simulink model "CCO_DSM_RDAC_02"  (R2021a)
settings: Solver=VariableStepAuto  StartTime=0.0  StopTime=6000*clk_p  RelTol=1e-3
values from neighbouring files (symbols this model uses):
  clk_p = 1/clk    (= 5e-09)    [parallel_simulink_test8.m]
  finw = 2*pi*M/(N_in*clk_p)    (= 3374757.73335)    [parallel_simulink_test8.m]
  N = 31    [GradientD_v6.m]    (also in N_selection.m = ceil(N); front_end_syn.m = input('How many stages of quantizer (enter num)? '); parallel_simulink_test8.m = 27; power_esti_v1.m)
  N_stage = N    (= 27)    [parallel_simulink_test8.m]
  Ph2 = circshift(Ph, (N_stage+1)/2)    [parallel_simulink_test8.m]
  Ru = VDD/(kdac*1e-6) - (Rcco*VDD*N)/(2*Amp) - N*Rcco    [solve_param_2nd.m]    (also in solve_param_2nd_1st.m; solve_param_RDAC_N_v5.m; solve_param_RDAC_N_v6.m; solve_param_comb_v1.m)
  S = 5    [GradientD_v6.m]    (also in parallel_simulink_test8.m; power_esti_v1.m; solve_param_2nd.m; solve_param_2nd_1st.m = 1)
  VDD = 1.2    [power_esti_v1.m]    (also in solve_param_2nd.m; solve_param_2nd_1st.m; solve_param_RDAC_N_v5.m; solve_param_RDAC_N_v6.m)
undefined symbols (not defined in the file or in its folder): Amp_in, Bias, Compen, fix_valid, gain_DAC, kcco_gain, Ph, Res, Res_CCO_fix
libraries: commblksprivate x4, simulink_extras x3, dspsigattribs x2, commsynccomp2 x2, simulink x1
settings Model: SimulationMode=accelerator  OrderedModelArguments=off  Creator=97826  LastModifiedBy=kli416
settings SolverCC: AlgebraicLoopSolver=LineSearch
settings DebuggingCC: SFMachineParentedDataDiag=warning
settings SFSimCC: CustomCodeUndefinedFunction=UseInterfaceOnly

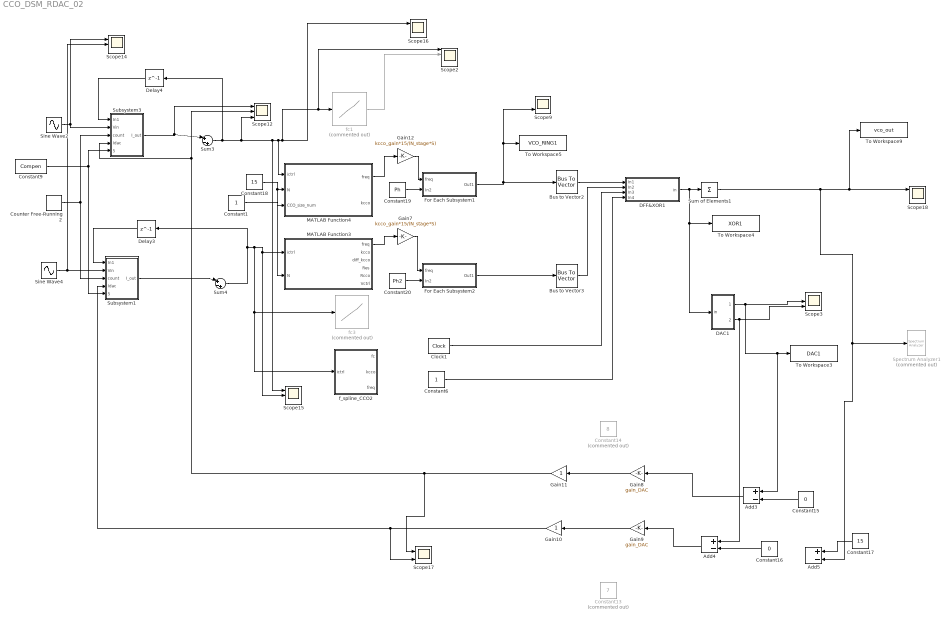
== system CCO_DSM_RDAC_02 ==
  Add3 : Sum  Inputs=+-
  Add4 : Sum  Inputs=+-
  Add5 : Sum  Inputs=+-
  Bus to Vector2 : BusToVector
  Bus to Vector3 : BusToVector
  Clock1 : simulink_extras/Flip Flops/Clock  period=clk_p
  Constant1 : Constant  VectorParams1D=off
  Constant13 : Constant  Commented=on  Value=7
  Constant14 : Constant  Commented=on  Value=8
  Constant15 : Constant  Value=0
  Constant16 : Constant  Value=0
  Constant17 : Constant  Value=15
  Constant18 : Constant  Value=15  VectorParams1D=off
  Constant19 : Constant  Value=Ph  VectorParams1D=off
  Constant20 : Constant  Value=Ph2  VectorParams1D=off
  Constant6 : Constant
  Constant9 : Constant  Value=Compen
  Counter Free-Running2 : simulink/Sources/Counter Free-Running  NumBits=32  tsamp=clk_p
  DAC1 : Subsystem
  DFF&XOR1 : Subsystem  TreatAsAtomicUnit=on
  Delay3 : Delay  DelayLength=1  SampleTime=clk_p
  Delay4 : Delay  DelayLength=1  SampleTime=clk_p
  For Each Subsystem1 : Subsystem  TreatAsAtomicUnit=on
  For Each Subsystem2 : Subsystem  TreatAsAtomicUnit=on
  Gain10 : Gain
  Gain11 : Gain
  Gain12 : Gain  Gain=kcco_gain*15/(N_stage*S)
  Gain7 : Gain  Gain=kcco_gain*15/(N_stage*S)
  Gain8 : Gain  Gain=gain_DAC
  Gain9 : Gain  Gain=gain_DAC
  MATLAB Function3 : MATLAB Function  TreatAsAtomicUnit=on
  MATLAB Function4 : MATLAB Function  TreatAsAtomicUnit=on
  Scope{3,12,14..16,18} (6 alike) : Scope  NumInputPorts=3
  Scope17 : Scope  NumInputPorts=2
  Scope2 : Scope  NumInputPorts=4
  Scope9 : Scope  NumInputPorts=2
  Sine Wave2 : Sin  Amplitude=Amp_in  Bias=Bias  Frequency=finw  SampleTime=0
  Sine Wave4 : Sin  Amplitude=Amp_in  Bias=Bias  Frequency=finw  Phase=pi  SampleTime=0
  Spectrum Analyzer1 : SpectrumAnalyzer  Commented=on
  Subsystem1 : Subsystem
  Subsystem3 : Subsystem
  Sum of Elements1 : Sum  Inputs=+  CollapseMode=Specified dimension
  Sum3 : Sum  Inputs=|+-+
  Sum4 : Sum  Inputs=|+-+
  To Workspace3 : ToWorkspace  VariableName=DAC1  SampleTime=-1
  To Workspace4 : ToWorkspace  VariableName=XOR1  SampleTime=-1
  To Workspace5 : ToWorkspace  VariableName=VCO_RING1  SampleTime=-1
  To Workspace9 : ToWorkspace  VariableName=vco_out  SampleTime=-1
  f_spline_CCO2 : MATLAB Function  TreatAsAtomicUnit=on
  fc1 : Lookup_n-D  Commented=on  NumberOfTableDimensions=1  BreakpointsForDimension1="[0.2, 0.3, 0.4, 0.5, 0.6, 0.7, 0.8, 0.9, 1.0, 1.1, 1.2, 1.3, 1.4, 1.5, 1.6, 1.7, 1.8, 1.9, 2, 3, 4, 5, 6, 7, 8, 9, 10, 15, 20, 25, 30, 35, 40, 45, 50, 55,  60, 65,  70, 75, 80, 85, 90, 95,  100, 105, 110, 115, 120, 125,  130, 135, 140, 145, 150, 155, 160, 165, 170, 175, 180, 185, 190, 195, 200]"  Table=|  InternalRulePriority=Speed  RndMeth=Simplest  InputSameDT=on
      | [1.66447511e+06, 2.39120610e+06, 3.09209814e+06, 3.77442525e+06,...
      |        4.44233187e+06, 5.09847708e+06, 5.74468330e+06, 6.38231333e+06,...
      |        7.01222933e+06, 7.63545294e+06, 8.25259544e+06, 8.86438379e+06,...
      |        9.47104229e+06, 1.00727251e+07, 1.06702063e+07, 1.12634810e+07,...
      |        1.18529335e+07, 1.24387856e+07, 1.30211555e+07, 1.86896325e+07,...
      |        2.41398372e+07, 2.94282099e+07, 3.45871163e+07, 3.96389683e+07,...
      |        4.45976622e+07, 4.94748247e+07, 5.42802707e+07, 7.74257487e+07,...
      |        9.94391631e+07, 1.20601948e+08, 1.41072774e+08, 1.60965277e+08,...
      |        1.80356637e+08, 1.99308797e+08, 2.17870620e+08, 2.36073995e+08,...
      |        2.53954710e+08, 2.71542852e+08, 2.88847872e+08, 3.05898332e+08,...
      |        3.22708688e+08, 3.39290137e+08, 3.55660515e+08, 3.71827383e+08,...
      |        3.87804329e+08, 4.03598484e+08, 4.19215145e+08, 4.34671106e+08,...
      |        4.49972102e+08, 4.65109789e+08, 4.80106776e+08, 4.94966194e+08,...
      |        5.09681398e+08, 5.24271132e+08, 5.38732148e+08, 5.53069814e+08,...
      |        5.67288983e+08, 5.81395349e+08, 5.95390487e+08, 6.09269425e+08,...
      |        6.23056841e+08, 6.36731783e+08, 6.50300764e+08, 6.63790242e+08,...
      |        6.77167274e+08]
  fc3 : Lookup_n-D  Commented=on  NumberOfTableDimensions=1  BreakpointsForDimension1="[0.2, 0.3, 0.4, 0.5, 0.6, 0.7, 0.8, 0.9, 1.0, 1.1, 1.2, 1.3, 1.4, 1.5, 1.6, 1.7, 1.8, 1.9, 2, 3, 4, 5, 6, 7, 8, 9, 10, 15, 20, 25, 30, 35, 40, 45, 50, 55,  60, 65,  70, 75, 80, 85, 90, 95,  100, 105, 110, 115, 120, 125,  130, 135, 140, 145, 150, 155, 160, 165, 170, 175, 180, 185, 190, 195, 200]"  Table=|  InternalRulePriority=Speed  RndMeth=Simplest  InputSameDT=on
      | [1.66447511e+06, 2.39120610e+06, 3.09209814e+06, 3.77442525e+06,...
      |        4.44233187e+06, 5.09847708e+06, 5.74468330e+06, 6.38231333e+06,...
      |        7.01222933e+06, 7.63545294e+06, 8.25259544e+06, 8.86438379e+06,...
      |        9.47104229e+06, 1.00727251e+07, 1.06702063e+07, 1.12634810e+07,...
      |        1.18529335e+07, 1.24387856e+07, 1.30211555e+07, 1.86896325e+07,...
      |        2.41398372e+07, 2.94282099e+07, 3.45871163e+07, 3.96389683e+07,...
      |        4.45976622e+07, 4.94748247e+07, 5.42802707e+07, 7.74257487e+07,...
      |        9.94391631e+07, 1.20601948e+08, 1.41072774e+08, 1.60965277e+08,...
      |        1.80356637e+08, 1.99308797e+08, 2.17870620e+08, 2.36073995e+08,...
      |        2.53954710e+08, 2.71542852e+08, 2.88847872e+08, 3.05898332e+08,...
      |        3.22708688e+08, 3.39290137e+08, 3.55660515e+08, 3.71827383e+08,...
      |        3.87804329e+08, 4.03598484e+08, 4.19215145e+08, 4.34671106e+08,...
      |        4.49972102e+08, 4.65109789e+08, 4.80106776e+08, 4.94966194e+08,...
      |        5.09681398e+08, 5.24271132e+08, 5.38732148e+08, 5.53069814e+08,...
      |        5.67288983e+08, 5.81395349e+08, 5.95390487e+08, 6.09269425e+08,...
      |        6.23056841e+08, 6.36731783e+08, 6.50300764e+08, 6.63790242e+08,...
      |        6.77167274e+08]
  wires:
  Delay3/1 -> Subsystem1/1(In1)
  Sine Wave2/1 -> Subsystem3/2(Vin), Scope14/1
  Add4/1 -> Gain9/1
  Gain12/1 -> For Each Subsystem1/1(freq)
  Constant9/1 -> Subsystem1/5(compen), Subsystem3/5(compen)
  Sum4/1 -> Delay3/1, Scope15/2, MATLAB Function3/1(ictrl), f_spline_CCO2/1(ictrl), fc3/1
  Delay4/1 -> Subsystem3/1(In1)
  Sum of Elements1/1 -> Spectrum Analyzer1/1, Add5/2, Scope18/1, To Workspace9/1
  Sum3/1 -> Delay4/1, Scope12/3, Scope15/1, MATLAB Function4/1(ictrl), Scope2/1, fc1/1, Scope16/1
  Subsystem3/1(I_out) -> Scope12/1, Sum3/1
  Constant19/1 -> For Each Subsystem1/2(In2)
  Bus to Vector2/1 -> DFF&XOR1/1(In1)
  fc1/1 -> Scope2/2
  Counter Free-Running2/1 -> Subsystem1/3(count), Subsystem3/3(count)
  DAC1/2(out2) -> Add4/1, Scope3/3
  Constant16/1 -> Add4/2
  Constant6/1 -> DFF&XOR1/4(In4)
  Gain8/1 -> Gain11/1
  Gain10/1 -> Subsystem1/4(Idac), Scope17/2
  Constant18/1 -> MATLAB Function3/2(N), MATLAB Function4/2(N)
  Gain7/1 -> For Each Subsystem2/1(freq)
  Constant17/1 -> Add5/1
  Constant20/1 -> For Each Subsystem2/2(In2)
  DAC1/1(out1) -> Add3/1, To Workspace3/1, Scope3/2
  Gain9/1 -> Gain10/1
  Clock1/1 -> DFF&XOR1/3(In3)
  Constant15/1 -> Add3/2
  DFF&XOR1/1(in) -> To Workspace4/1, DAC1/1(in), Sum of Elements1/1
  Subsystem1/1(I_out) -> Sum4/1
  Bus to Vector3/1 -> DFF&XOR1/2(In2)
  For Each Subsystem2/1(Out1) -> Bus to Vector3/1
  Sine Wave4/1 -> Subsystem1/2(Vin), Scope14/2
  For Each Subsystem1/1(Out1) -> To Workspace5/1, Scope9/2, Bus to Vector2/1
  Add3/1 -> Gain8/1
  Gain11/1 -> Subsystem3/4(Idac), Scope12/2, Scope17/1
  MATLAB Function3/1(freq) -> Gain7/1
  MATLAB Function4/1(freq) -> Gain12/1
  Constant1/1 -> MATLAB Function4/3(CCO_size_num)

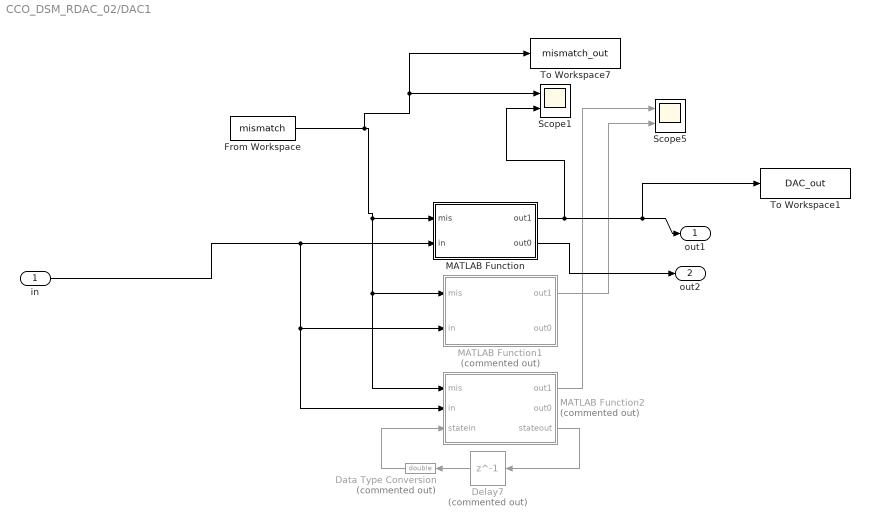
== system CCO_DSM_RDAC_02/DAC1 ==
  in : Inport
  Data Type Conversion : DataTypeConversion  Commented=on  OutDataTypeStr=double
  Delay7 : Delay  Commented=on  DelayLength=1  SampleTime=clk_p
  From Workspace : FromWorkspace  VariableName=mismatch
  MATLAB Function : MATLAB Function  TreatAsAtomicUnit=on
  MATLAB Function1 : MATLAB Function  Commented=on  TreatAsAtomicUnit=on
  MATLAB Function2 : MATLAB Function  Commented=on  TreatAsAtomicUnit=on
  Scope1 : Scope  NumInputPorts=2
  Scope5 : Scope  NumInputPorts=2
  To Workspace1 : ToWorkspace  VariableName=DAC_out  SampleTime=-1
  To Workspace7 : ToWorkspace  VariableName=mismatch_out  SampleTime=-1
  out1 : Outport
  out2 : Outport  Port=2
  wires:
  From Workspace/1 -> To Workspace7/1, Scope1/1, MATLAB Function2/1(mis), MATLAB Function1/1(mis), MATLAB Function/1(mis)
  MATLAB Function1/1(out1) -> Scope5/2
  MATLAB Function2/1(out1) -> Scope5/1
  MATLAB Function2/3(stateout) -> Delay7/1
  Delay7/1 -> Data Type Conversion/1
  Data Type Conversion/1 -> MATLAB Function2/3(statein)
  MATLAB Function/1(out1) -> Scope1/2, To Workspace1/1, out1/1
  MATLAB Function/2(out0) -> out2/1
  in/1 -> MATLAB Function2/2(in), MATLAB Function1/2(in), MATLAB Function/2(in)

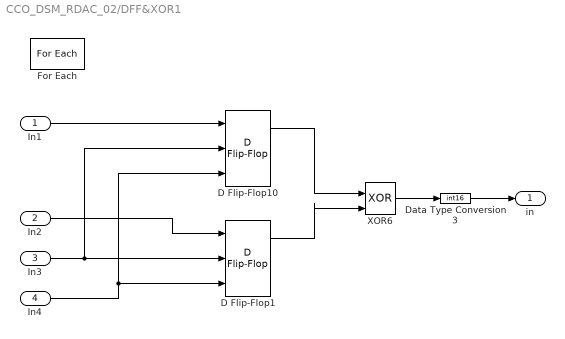
== system CCO_DSM_RDAC_02/DFF&XOR1 ==
  In1 : Inport  Partition=on  PartitionDimension=1  PartitionWidth=N_stage  PartitionOffset=0
  In2 : Inport  Port=2  Partition=on  PartitionDimension=1  PartitionWidth=N_stage  PartitionOffset=0
  In3 : Inport  Port=3
  In4 : Inport  Port=4
  D Flip-Flop1 : simulink_extras/Flip Flops/D Flip-Flop
  D Flip-Flop10 : simulink_extras/Flip Flops/D Flip-Flop
  Data Type Conversion3 : DataTypeConversion  OutDataTypeStr=int16
  For Each : ForEach  DisableCoverage=on
  XOR6 : Logic  Operator=XOR  IconShape=distinctive  AllPortsSameDT=off  OutDataTypeStr=boolean
  in : Outport  ConcatenationDimension=1
  wires:
  In1/1 -> D Flip-Flop10/1
  In3/1 -> D Flip-Flop1/2, D Flip-Flop10/2
  In4/1 -> D Flip-Flop1/3, D Flip-Flop10/3
  In2/1 -> D Flip-Flop1/1
  D Flip-Flop10/1 -> XOR6/1
  D Flip-Flop1/1 -> XOR6/2
  XOR6/1 -> Data Type Conversion3/1
  Data Type Conversion3/1 -> in/1

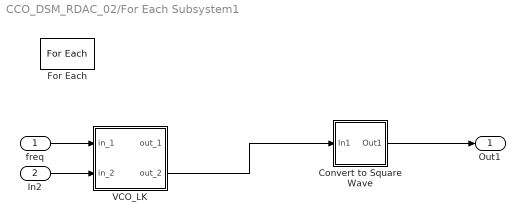
== system CCO_DSM_RDAC_02/For Each Subsystem1 ==
  freq : Inport
  In2 : Inport  Port=2  Partition=on  PartitionDimension=1  PartitionWidth=1  PartitionOffset=0
  Convert to Square Wave : Subsystem
  For Each : ForEach  DisableCoverage=on
  VCO_LK : Subsystem  mask{Ac=1, Fc=1, Kc=1, Ph=1}
  Out1 : Outport  ConcatenationDimension=1
  wires:
  freq/1 -> VCO_LK/1(in_1)
  Convert to Square Wave/1(Out1) -> Out1/1
  VCO_LK/2(out_2) -> Convert to Square Wave/1(In1)
  In2/1 -> VCO_LK/2(in_2)

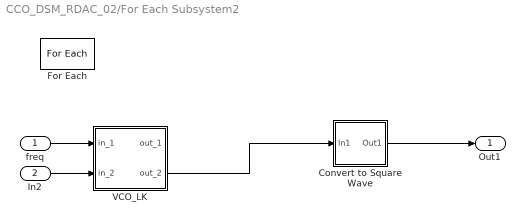
== system CCO_DSM_RDAC_02/For Each Subsystem2 ==
  freq : Inport
  In2 : Inport  Port=2  Partition=on  PartitionDimension=1  PartitionWidth=1  PartitionOffset=0
  Convert to Square Wave : Subsystem
  For Each : ForEach  DisableCoverage=on
  VCO_LK : Subsystem  mask{Ac=1, Fc=1, Kc=1, Ph=1}
  Out1 : Outport  ConcatenationDimension=1
  wires:
  freq/1 -> VCO_LK/1(in_1)
  Convert to Square Wave/1(Out1) -> Out1/1
  VCO_LK/2(out_2) -> Convert to Square Wave/1(In1)
  In2/1 -> VCO_LK/2(in_2)

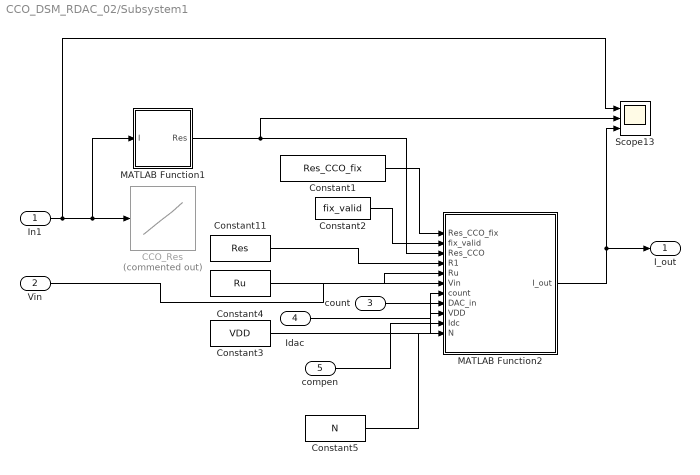
== system CCO_DSM_RDAC_02/Subsystem1 ==
  In1 : Inport
  Vin : Inport  Port=2
  count : Inport  Port=3
  Idac : Inport  Port=4
  compen : Inport  Port=5
  CCO_Res : Lookup_n-D  Commented=on  NumberOfTableDimensions=1  BreakpointsForDimension1="[0.2, 0.3, 0.4, 0.5, 0.6, 0.7, 0.8, 0.9, 1.0, 1.1, 1.2, 1.3, 1.4, 1.5, 1.6, 1.7, 1.8, 1.9, 2, 3, 4, 5, 6, 7, 8, 9, 10, 15, 20, 25, 30, 35, 40, 45, 50, 55,  60, 65,  70, 75, 80, 85, 90, 95,  100, 105, 110, 115, 120, 125,  130, 135, 140, 145, 150, 155, 160, 165, 170, 175, 180, 185, 190, 195, 200]"  Table=|  InternalRulePriority=Speed  RndMeth=Simplest  InputSameDT=on
      | [1537660.  , 1077280.  ,  842821.  ,  698885.  ,  591175.  ,...
      |         514638.  ,  459534.  ,  412343.  ,  375823.  ,  346689.  ,...
      |         319079.  ,  297528.  ,  279608.  ,  262772.  ,  247488.  ,...
      |         234050.  ,  222561.  ,  212364.  ,  203057.  ,  141281.  ,...
      |         109313.  ,   89599.1 ,   76189.9 ,   66472.9 ,   58960.7 ,...
      |          53105.2 ,   48293.7 ,   33792.1 ,   26194.2 ,   21517.8 ,...
      |          18368.6 ,   16013.  ,   14184.9 ,   12812.5 ,   11686.2 ,...
      |          10767.2 ,    9950.94,    9274.88,    8702.95,    8196.31,...
      |           7752.34,    7370.14,    7028.82,    6691.36,    6410.4 ,...
      |           6146.98,    5908.61,    5682.79,    5493.1 ,    5296.82,...
      |           5117.51,    4962.31,    4815.99,    4677.93,    4545.02,...
      |           4420.64,    4304.52,    4195.05,    4089.12,    3988.32,...
      |           3892.26,    3805.99,    3726.36,    3645.09,    3564.56]
  Constant1 : Constant  Value=Res_CCO_fix
  Constant11 : Constant  Value=Res
  Constant2 : Constant  Value=fix_valid
  Constant3 : Constant  Value=VDD
  Constant4 : Constant  Value=Ru
  Constant5 : Constant  Value=N
  MATLAB Function1 : MATLAB Function  TreatAsAtomicUnit=on
  MATLAB Function2 : MATLAB Function  TreatAsAtomicUnit=on
  Scope13 : Scope  NumInputPorts=3
  I_out : Outport
  wires:
  Constant11/1 -> MATLAB Function2/4(R1)
  Vin/1 -> MATLAB Function2/6(Vin)
  In1/1 -> MATLAB Function1/1(I), CCO_Res/1, Scope13/1
  MATLAB Function2/1(I_out) -> Scope13/3, I_out/1
  count/1 -> MATLAB Function2/7(count)
  Constant1/1 -> MATLAB Function2/1(Res_CCO_fix)
  Constant2/1 -> MATLAB Function2/2(fix_valid)
  MATLAB Function1/1(Res) -> MATLAB Function2/3(Res_CCO), Scope13/2
  compen/1 -> MATLAB Function2/10(Idc)
  Constant3/1 -> MATLAB Function2/9(VDD)
  Idac/1 -> MATLAB Function2/8(DAC_in)
  Constant4/1 -> MATLAB Function2/5(Ru)
  Constant5/1 -> MATLAB Function2/11(N)

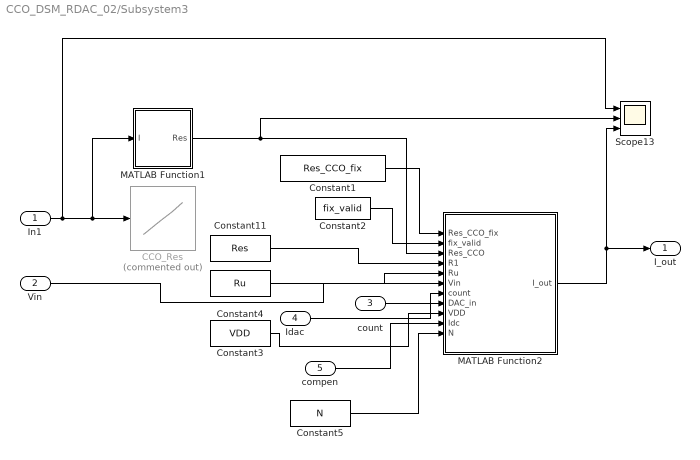
== system CCO_DSM_RDAC_02/Subsystem3 ==
  In1 : Inport
  Vin : Inport  Port=2
  count : Inport  Port=3
  Idac : Inport  Port=4
  compen : Inport  Port=5
  CCO_Res : Lookup_n-D  Commented=on  NumberOfTableDimensions=1  BreakpointsForDimension1="[0.2, 0.3, 0.4, 0.5, 0.6, 0.7, 0.8, 0.9, 1.0, 1.1, 1.2, 1.3, 1.4, 1.5, 1.6, 1.7, 1.8, 1.9, 2, 3, 4, 5, 6, 7, 8, 9, 10, 15, 20, 25, 30, 35, 40, 45, 50, 55,  60, 65,  70, 75, 80, 85, 90, 95,  100, 105, 110, 115, 120, 125,  130, 135, 140, 145, 150, 155, 160, 165, 170, 175, 180, 185, 190, 195, 200]"  Table=|  InternalRulePriority=Speed  RndMeth=Simplest  InputSameDT=on
      | [1537660.  , 1077280.  ,  842821.  ,  698885.  ,  591175.  ,...
      |         514638.  ,  459534.  ,  412343.  ,  375823.  ,  346689.  ,...
      |         319079.  ,  297528.  ,  279608.  ,  262772.  ,  247488.  ,...
      |         234050.  ,  222561.  ,  212364.  ,  203057.  ,  141281.  ,...
      |         109313.  ,   89599.1 ,   76189.9 ,   66472.9 ,   58960.7 ,...
      |          53105.2 ,   48293.7 ,   33792.1 ,   26194.2 ,   21517.8 ,...
      |          18368.6 ,   16013.  ,   14184.9 ,   12812.5 ,   11686.2 ,...
      |          10767.2 ,    9950.94,    9274.88,    8702.95,    8196.31,...
      |           7752.34,    7370.14,    7028.82,    6691.36,    6410.4 ,...
      |           6146.98,    5908.61,    5682.79,    5493.1 ,    5296.82,...
      |           5117.51,    4962.31,    4815.99,    4677.93,    4545.02,...
      |           4420.64,    4304.52,    4195.05,    4089.12,    3988.32,...
      |           3892.26,    3805.99,    3726.36,    3645.09,    3564.56]
  Constant1 : Constant  Value=Res_CCO_fix
  Constant11 : Constant  Value=Res
  Constant2 : Constant  Value=fix_valid
  Constant3 : Constant  Value=VDD
  Constant4 : Constant  Value=Ru
  Constant5 : Constant  Value=N
  MATLAB Function1 : MATLAB Function  TreatAsAtomicUnit=on
  MATLAB Function2 : MATLAB Function  TreatAsAtomicUnit=on
  Scope13 : Scope  NumInputPorts=3
  I_out : Outport
  wires:
  Constant11/1 -> MATLAB Function2/4(R1)
  Vin/1 -> MATLAB Function2/6(Vin)
  In1/1 -> MATLAB Function1/1(I), CCO_Res/1, Scope13/1
  MATLAB Function2/1(I_out) -> Scope13/3, I_out/1
  count/1 -> MATLAB Function2/7(count)
  Constant1/1 -> MATLAB Function2/1(Res_CCO_fix)
  Constant2/1 -> MATLAB Function2/2(fix_valid)
  MATLAB Function1/1(Res) -> MATLAB Function2/3(Res_CCO), Scope13/2
  compen/1 -> MATLAB Function2/10(Idc)
  Constant3/1 -> MATLAB Function2/9(VDD)
  Idac/1 -> MATLAB Function2/8(DAC_in)
  Constant4/1 -> MATLAB Function2/5(Ru)
  Constant5/1 -> MATLAB Function2/11(N)

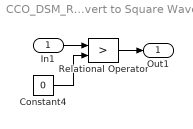
== system CCO_DSM_RDAC_02/For Each Subsystem1/Convert to Square Wave ==
  In1 : Inport
  Constant4 : Constant  Value=0
  Relational Operator : RelationalOperator  Operator=>  RndMeth=Nearest  InputSameDT=on
  Out1 : Outport
  wires:
  Relational Operator/1 -> Out1/1
  In1/1 -> Relational Operator/1
  Constant4/1 -> Relational Operator/2

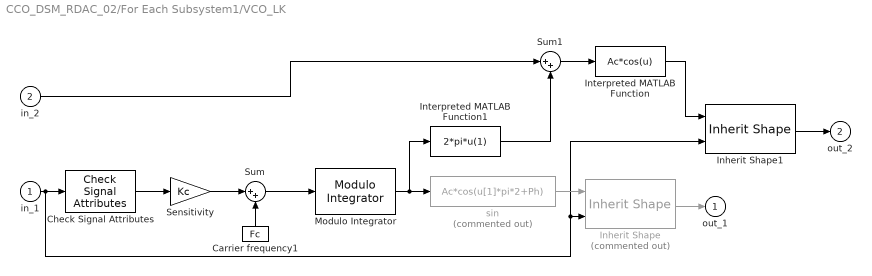
== system CCO_DSM_RDAC_02/For Each Subsystem1/VCO_LK ==
  in_1 : Inport
  in_2 : Inport  Port=2
  Carrier frequency1 : Constant  Value=Fc
  Check Signal Attributes : dspsigattribs/Check Signal Attributes  SigAttribCheckMethod=Does not match attributes exactly  Complexity=Ignore  Frame=Sample-based  DimsCheckMethod=Ignore  Dimensions=Vector (1-D or 2-D) or scalar  DatatypeCheckMethod=Ignore  DatatypeGeneral=Floating-point  DtypeFloatSpecific=Double precision  DtypeFixedSpecific=Any fixed-point  DtypeIntSpecific=Any integer  SampleMode=Ignore
      settings: SourceProductName=DSP System Toolbox
  Inherit Shape : commblksprivate/Inherit Shape  Commented=on
      settings: SourceProductBaseCode=CM
  Inherit Shape1 : commblksprivate/Inherit Shape
      settings: SourceProductBaseCode=CM
  Interpreted MATLAB Function : MATLABFcn  MATLABFcn=Ac*cos(u)
  Interpreted MATLAB Function1 : MATLABFcn  MATLABFcn=2*pi*u(1)
  Modulo Integrator : commsynccomp2/Continuous-Time VCO/Modulo  Integrator  SystemSampleTime=-1
      settings: SourceProductBaseCode=CM
  Sensitivity : Gain  Gain=Kc  SaturateOnIntegerOverflow=on  OutDataTypeStr=Inherit: Same as input  ParamDataTypeStr=Inherit: Same as input
  Sum : Sum  Inputs=|++  InputSameDT=on  SaturateOnIntegerOverflow=on  OutDataTypeStr=Inherit: Same as first input
  Sum1 : Sum  Inputs=|++  InputSameDT=on  SaturateOnIntegerOverflow=on  OutDataTypeStr=Inherit: Same as first input
  sin : Fcn  Commented=on  Expr=Ac*cos(u[1]*pi*2+Ph)
  out_1 : Outport  InitialOutput=0  VectorParamsAs1DForOutWhenUnconnected=off
  out_2 : Outport  Port=2  InitialOutput=0  VectorParamsAs1DForOutWhenUnconnected=off
  wires:
  Sum/1 -> Modulo Integrator/1
  Modulo Integrator/1 -> Interpreted MATLAB Function1/1, sin/1
  Carrier frequency1/1 -> Sum/2
  Inherit Shape/1 -> out_1/1
  Check Signal Attributes/1 -> Sensitivity/1
  in_1/1 -> Check Signal Attributes/1, Inherit Shape1/2, Inherit Shape/2
  sin/1 -> Inherit Shape/1
  Sensitivity/1 -> Sum/1
  in_2/1 -> Sum1/1
  Sum1/1 -> Interpreted MATLAB Function/1
  Interpreted MATLAB Function1/1 -> Sum1/2
  Interpreted MATLAB Function/1 -> Inherit Shape1/1
  Inherit Shape1/1 -> out_2/1

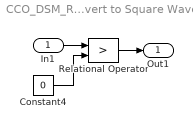
== system CCO_DSM_RDAC_02/For Each Subsystem2/Convert to Square Wave ==
  In1 : Inport
  Constant4 : Constant  Value=0
  Relational Operator : RelationalOperator  Operator=>  RndMeth=Nearest  InputSameDT=on
  Out1 : Outport
  wires:
  Relational Operator/1 -> Out1/1
  In1/1 -> Relational Operator/1
  Constant4/1 -> Relational Operator/2

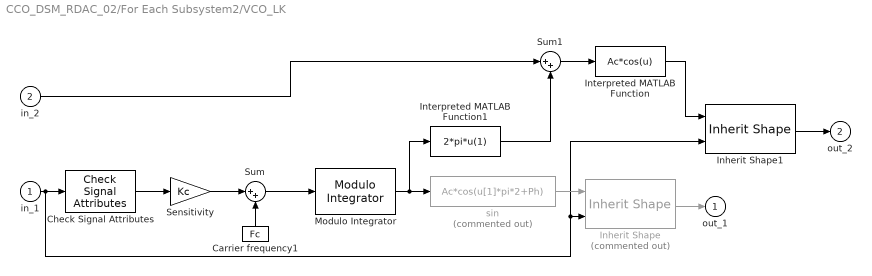
== system CCO_DSM_RDAC_02/For Each Subsystem2/VCO_LK ==
  in_1 : Inport
  in_2 : Inport  Port=2
  Carrier frequency1 : Constant  Value=Fc
  Check Signal Attributes : dspsigattribs/Check Signal Attributes  SigAttribCheckMethod=Does not match attributes exactly  Complexity=Ignore  Frame=Sample-based  DimsCheckMethod=Ignore  Dimensions=Vector (1-D or 2-D) or scalar  DatatypeCheckMethod=Ignore  DatatypeGeneral=Floating-point  DtypeFloatSpecific=Double precision  DtypeFixedSpecific=Any fixed-point  DtypeIntSpecific=Any integer  SampleMode=Ignore
      settings: SourceProductName=DSP System Toolbox
  Inherit Shape : commblksprivate/Inherit Shape  Commented=on
      settings: SourceProductBaseCode=CM
  Inherit Shape1 : commblksprivate/Inherit Shape
      settings: SourceProductBaseCode=CM
  Interpreted MATLAB Function : MATLABFcn  MATLABFcn=Ac*cos(u)
  Interpreted MATLAB Function1 : MATLABFcn  MATLABFcn=2*pi*u(1)
  Modulo Integrator : commsynccomp2/Continuous-Time VCO/Modulo  Integrator  SystemSampleTime=-1
      settings: SourceProductBaseCode=CM
  Sensitivity : Gain  Gain=Kc  SaturateOnIntegerOverflow=on  OutDataTypeStr=Inherit: Same as input  ParamDataTypeStr=Inherit: Same as input
  Sum : Sum  Inputs=|++  InputSameDT=on  SaturateOnIntegerOverflow=on  OutDataTypeStr=Inherit: Same as first input
  Sum1 : Sum  Inputs=|++  InputSameDT=on  SaturateOnIntegerOverflow=on  OutDataTypeStr=Inherit: Same as first input
  sin : Fcn  Commented=on  Expr=Ac*cos(u[1]*pi*2+Ph)
  out_1 : Outport  InitialOutput=0  VectorParamsAs1DForOutWhenUnconnected=off
  out_2 : Outport  Port=2  InitialOutput=0  VectorParamsAs1DForOutWhenUnconnected=off
  wires:
  Sum/1 -> Modulo Integrator/1
  Modulo Integrator/1 -> Interpreted MATLAB Function1/1, sin/1
  Carrier frequency1/1 -> Sum/2
  Inherit Shape/1 -> out_1/1
  Check Signal Attributes/1 -> Sensitivity/1
  in_1/1 -> Check Signal Attributes/1, Inherit Shape1/2, Inherit Shape/2
  sin/1 -> Inherit Shape/1
  Sensitivity/1 -> Sum/1
  in_2/1 -> Sum1/1
  Sum1/1 -> Interpreted MATLAB Function/1
  Interpreted MATLAB Function1/1 -> Sum1/2
  Interpreted MATLAB Function/1 -> Inherit Shape1/1
  Inherit Shape1/1 -> out_2/1

== matlab function CCO_DSM_RDAC_02/Subsystem3/MATLAB Function2 ==
  data: Res_CCO_fix input; fix_valid input; Res_CCO input; I_out output; R1 input; Ru input; Vin input; count input; DAC_in input; VDD input; Idc input; N input
function I_out = current(Res_CCO_fix, fix_valid, Res_CCO, R1, Ru, Vin, count, DAC_in, VDD, Idc, N)
if (fix_valid == 1)
    %I_out = (Vin-(Idac-compen)*Res*1e-6)/(Res_CCO_fix + Res)*1e6;
    I_out = (Vin/R1*1e6+DAC_in*VDD/Ru*1e6+Idc)/(1+Res_CCO_fix/R1+Res_CCO_fix*N/Ru);
else
    if (count>5)
        I_out = (Vin/R1*1e6+DAC_in*VDD/Ru*1e6+Idc)/(1+Res_CCO/R1+Res_CCO*N/Ru);
    else
        I_out = (Vin/R1*1e6+DAC_in*VDD/Ru*1e6+Idc)/(1+Res_CCO_fix/R1+Res_CCO_fix*N/Ru);
    end
%165e3  47e3  57e3
end
end

== matlab function CCO_DSM_RDAC_02/f_spline_CCO2 ==
  data: fc output; ictrl input; kcco output; freq output
function [fc, kcco,freq]=f_spline_CCO(ictrl)
delta = 0.0001; % use to calc kvco
gamma = 0.1;
x = [0.2, 0.3, 0.4, 0.5, 0.6, 0.7, 0.8, 0.9, 1.0, 1.1, 1.2, 1.3, 1.4, 1.5, 1.6, 1.7, 1.8, 1.9, 2, 3, 4, 5, 6, 7, 8, 9, 10, 15, 20, 25, 30, 35, 40, 45, 50, 55,  60, 65,  70, 75, 80, 85, 90, 95,  100, 105, 110, 115, 120, 125,  130, 135, 140, 145, 150, 155, 160, 165, 170, 175, 180, 185, 190, 195, 200];
freq_0f = 	[1.66447511e+06, 2.39120610e+06, 3.09209814e+06, 3.77442525e+06,...
       4.44233187e+06, 5.09847708e+06, 5.74468330e+06, 6.38231333e+06,...
       7.01222933e+06, 7.63545294e+06, 8.25259544e+06, 8.86438379e+06,...
       9.47104229e+06, 1.00727251e+07, 1.06702063e+07, 1.12634810e+07,...
       1.18529335e+07, 1.24387856e+07, 1.30211555e+07, 1.86896325e+07,...
       2.41398372e+07, 2.94282099e+07, 3.45871163e+07, 3.96389683e+07,...
       4.45976622e+07, 4.94748247e+07, 5.42802707e+07, 7.74257487e+07,...
       9.94391631e+07, 1.20601948e+08, 1.41072774e+08, 1.60965277e+08,...
       1.80356637e+08, 1.99308797e+08, 2.17870620e+08, 2.36073995e+08,...
       2.53954710e+08, 2.71542852e+08, 2.88847872e+08, 3.05898332e+08,...
       3.22708688e+08, 3.39290137e+08, 3.55660515e+08, 3.71827383e+08,...
       3.87804329e+08, 4.03598484e+08, 4.19215145e+08, 4.34671106e+08,...
       4.49972102e+08, 4.65109789e+08, 4.80106776e+08, 4.94966194e+08,...
       5.09681398e+08, 5.24271132e+08, 5.38732148e+08, 5.53069814e+08,...
       5.67288983e+08, 5.81395349e+08, 5.95390487e+08, 6.09269425e+08,...
       6.23056841e+08, 6.36731783e+08, 6.50300764e+08, 6.63790242e+08,...
       6.77167274e+08];
%freq = spline(x(1:10),freq_0f(1:10),ictrl);  
fc = spline(x,freq_0f,ictrl);
kcco = (spline(x,freq_0f,ictrl+delta/2)-spline(x,freq_0f,ictrl-delta/2))/delta;
%diff_kcco = ((spline(x,freq_0f,ictrl+delta/2+gamma/2)-spline(x,freq_0f,ictrl-delta/2+gamma/2))/delta-(spline(x,freq_0f,ictrl+delta/2-gamma/2)-spline(x,freq_0f,ictrl-delta/2-gamma/2))/delta)/gamma;
freq = kcco*ictrl + fc;
end

== matlab function CCO_DSM_RDAC_02/DAC1/MATLAB Function ==
  data: mis input; out1 output; in input; out0 output
function [out1, out0]= DAC_CLA(mis, in)
out1 = 0;
out0 = 0;
b = size(mis);
t = b(1);
for i = 1:t %15
    if (in(i)==1)
        out1 = out1 + mis(i);
    else
        out0 = out0 + mis(i);
    end
end
end

== matlab function CCO_DSM_RDAC_02/DAC1/MATLAB Function1 ==
  data: mis input; out1 output; in input; out0 output
function [out1, out0]= DAC_thermo(mis, in)
out1 = 0;
out0 = 0;
sum = int16(0);
sum_mis = 0;

for i = 1:15
    sum = sum + in(i);
    sum_mis= sum_mis + mis(i);
end

for j = 1:sum
    out1 = out1 + mis(j);
end

out0 = sum_mis - out1;
end

== matlab function CCO_DSM_RDAC_02/DAC1/MATLAB Function2 ==
  data: mis input; out1 output; in input; out0 output; statein input; stateout output
function [out1, out0, stateout]= DAC_DWA(mis, in,statein)
enable = 1;
out1 = 0;
out0 = 0;
data = int16(0);

bitout=zeros(15,1);

for i = 1:15
    data = data + in(i);
end


stateplus=data;
if enable==0;
    stateout=statein;
else
    stateout=statein+stateplus;
end

if (stateout>14)
    stateout=stateout-15;
end

for i=15:-1:1
    if (stateout+data<15)
        if (i<stateout+1 || i>(stateout+data))
        bitout(i)=0;
        else
            bitout(i)=1;
        end
    else
        if (i>stateout || i<(stateout+data-14))
        bitout(i)=1;
        else
            bitout(i)=0;
        end
    end
end

for i = 1:15
    if (bitout(i)==1)
        out1 = out1 + mis(i);
    else
        out0 = out0 + mis(i);
    end
end

end

== matlab function CCO_DSM_RDAC_02/MATLAB Function3 ==
  data: ictrl input; freq output; N input; kcco output; diff_kcco output; Res output; Rcco output; Vctrl output
%12/07/2021
%0.2uA to 500uA, 15 stages

function [freq, kcco,diff_kcco, Res, Rcco, Vctrl]=f_spline_CCO_all_size_v2(ictrl,N)
%%%%%test func
%ictrl = 200;
%N = 31;
CCO_size = "CCO82_0f";
%%%%%

delta = 0.0001; % use to calc kvco
gamma = 0.1;

Delay_CCO82 = load('/nethome/kli416/Downloads/VCO/Work/CCO_size_result/Delay_CCO_ring82.txt');
Delay_CCO124 = load('/nethome/kli416/Downloads/VCO/Work/CCO_size_result/Delay_CCO_ring124.txt');
Delay_CCO164 = load('/nethome/kli416/Downloads/VCO/Work/CCO_size_result/Delay_CCO_ring164.txt');
Delay_CCO206 = load('/nethome/kli416/Downloads/VCO/Work/CCO_size_result/Delay_CCO_ring206.txt');
Delay_CCO248 = load('/nethome/kli416/Downloads/VCO/Work/CCO_size_result/Delay_CCO_ring248.txt');
x = [0.2, 0.3, 0.4, 0.5, 0.6, 0.7, 0.8, 0.9, 1.0, 1.1, 1.2, 1.3, 1.4, 1.5, 1.6, 1.7, 1.8, 1.9, 2, 3, 4, 5, 6, 7, 8, 9, 10, 15, 20, 25, 30, 35, 40, 45, 50, 55,  60, 65,  70, 75, 80, 85, 90, 95,  100, 105, 110, 115, 120, 125,  130, 135, 140, 145, 150, 155, 160, 165, 170, 175, 180, 185, 190, 195, 200, 210, 220, 230, 240, 250, 260, 270, 280, 290, 300, 310, 320, 330, 340, 350, 360, 370, 380, 390, 400, 410, 420, 430, 440, 450, 460, 470, 480, 490, 500];
size_x = size(x);
freq_sel = zeros(size_x(2),1);

freq_CCO82_15S_0f = 1./Delay_CCO82(:,1);
freq_CCO82_0f = freq_CCO82_15S_0f*15/N;
freq_CCO82_15S_10f = 1./Delay_CCO82(:,4);
freq_CCO82_10f = freq_CCO82_15S_10f*15/N;
freq_CCO82_15S_20f = 1./Delay_CCO82(:,7);
freq_CCO82_20f = freq_CCO82_15S_20f*15/N;

Res_CCO82_15S_0f = Delay_CCO82(:,3);
Res_CCO82_0f = Res_CCO82_15S_0f;
Res_CCO82_15S_10f = Delay_CCO82(:,6);
Res_CCO82_10f = Res_CCO82_15S_10f;
Res_CCO82_15S_20f = Delay_CCO82(:,9);
Res_CCO82_20f = Res_CCO82_15S_20f;

Vol_CCO82_0f = Delay_CCO82(:,2);
Vol_CCO82_10f = Delay_CCO82(:,5);
Vol_CCO82_20f = Delay_CCO82(:,8);


freq_CCO124_15S_0f = 1./Delay_CCO124(:,1);
freq_CCO124_0f = freq_CCO124_15S_0f*15/N;
freq_CCO124_15S_10f = 1./Delay_CCO124(:,4);
freq_CCO124_10f = freq_CCO124_15S_10f*15/N;
freq_CCO124_15S_20f = 1./Delay_CCO124(:,7);
freq_CCO124_20f = freq_CCO124_15S_20f*15/N;

Res_CCO124_15S_0f = Delay_CCO124(:,3);
Res_CCO124_0f = Res_CCO124_15S_0f;
Res_CCO124_15S_10f = Delay_CCO124(:,6);
Res_CCO124_10f = Res_CCO124_15S_10f;
Res_CCO124_15S_20f = Delay_CCO124(:,9);
Res_CCO124_20f = Res_CCO124_15S_20f;

Vol_CCO124_0f = Delay_CCO124(:,2);
Vol_CCO124_10f = Delay_CCO124(:,5);
Vol_CCO124_20f = Delay_CCO124(:,8);


freq_CCO164_15S_0f = 1./Delay_CCO164(:,1);
freq_CCO164_0f = freq_CCO164_15S_0f*15/N;
freq_CCO164_15S_10f = 1./Delay_CCO164(:,4);
freq_CCO164_10f = freq_CCO164_15S_10f*15/N;
freq_CCO164_15S_20f = 1./Delay_CCO164(:,7);
freq_CCO164_20f = freq_CCO164_15S_20f*15/N;

Res_CCO164_15S_0f = Delay_CCO164(:,3);
Res_CCO164_0f = Res_CCO164_15S_0f;
Res_CCO164_15S_10f = Delay_CCO164(:,6);
Res_CCO164_10f = Res_CCO164_15S_10f;
Res_CCO164_15S_20f = Delay_CCO164(:,9);
Res_CCO164_20f = Res_CCO164_15S_20f;

Vol_CCO164_0f = Delay_CCO164(:,2);
Vol_CCO164_10f = Delay_CCO164(:,5);
Vol_CCO164_20f = Delay_CCO164(:,8);


freq_CCO206_15S_0f = 1./Delay_CCO206(:,1);
freq_CCO206_0f = freq_CCO206_15S_0f*15/N;
freq_CCO206_15S_10f = 1./Delay_CCO206(:,4);
freq_CCO206_10f = freq_CCO206_15S_10f*15/N;
freq_CCO206_15S_20f = 1./Delay_CCO206(:,7);
freq_CCO206_20f = freq_CCO206_15S_20f*15/N;

Res_CCO206_15S_0f = Delay_CCO206(:,3);
Res_CCO206_0f = Res_CCO206_15S_0f;
Res_CCO206_15S_10f = Delay_CCO206(:,6);
Res_CCO206_10f = Res_CCO206_15S_10f;
Res_CCO206_15S_20f = Delay_CCO206(:,9);
Res_CCO206_20f = Res_CCO206_15S_20f;

Vol_CCO206_0f = Delay_CCO206(:,2);
Vol_CCO206_10f = Delay_CCO206(:,5);
Vol_CCO206_20f = Delay_CCO206(:,8);


freq_CCO248_15S_0f = 1./Delay_CCO248(:,1);
freq_CCO248_0f = freq_CCO248_15S_0f*15/N;
freq_CCO248_15S_10f = 1./Delay_CCO248(:,4);
freq_CCO248_10f = freq_CCO248_15S_10f*15/N;
freq_CCO248_15S_20f = 1./Delay_CCO248(:,7);
freq_CCO248_20f = freq_CCO248_15S_20f*15/N;

Res_CCO248_15S_0f = Delay_CCO248(:,3);
Res_CCO248_0f = Res_CCO248_15S_0f;
Res_CCO248_15S_10f = Delay_CCO248(:,6);
Res_CCO248_10f = Res_CCO248_15S_10f;
Res_CCO248_15S_20f = Delay_CCO248(:,9);
Res_CCO248_20f = Res_CCO248_15S_20f;

Vol_CCO248_0f = Delay_CCO248(:,2);
Vol_CCO248_10f = Delay_CCO248(:,5);
Vol_CCO248_20f = Delay_CCO248(:,8);


switch(CCO_size)
    case "CCO82_0f"
        freq_sel = freq_CCO82_0f;
        Res_sel = Res_CCO82_0f;
        Vol_sel = Vol_CCO82_0f;
    case "CCO82_10f"
        freq_sel = freq_CCO82_10f;
        Res_sel = Res_CCO82_10f;
        Vol_sel = Vol_CCO82_10f;
    case "CCO82_20f"
        freq_sel = freq_CCO82_20f;
        Res_sel = Res_CCO82_20f;
        Vol_sel = Vol_CCO82_20f;
    case "CCO124_0f"
        freq_sel = freq_CCO124_0f;
        Res_sel = Res_CCO124_0f;
        Vol_sel = Vol_CCO124_0f;
    case "CCO124_10f"
        freq_sel = freq_CCO124_10f;
        Res_sel = Res_CCO124_10f;
        Vol_sel = Vol_CCO124_10f;
    case "CCO124_20f"
        freq_sel = freq_CCO124_20f;
        Res_sel = Res_CCO124_20f;
        Vol_sel = Vol_CCO124_20f;
    case "CCO164_0f"
        freq_sel = freq_CCO164_0f;
        Res_sel = Res_CCO164_0f;
        Vol_sel = Vol_CCO164_0f;
    case "CCO164_10f"
        freq_sel = freq_CCO164_10f;
        Res_sel = Res_CCO164_10f;
        Vol_sel = Vol_CCO164_10f;
    case "CCO164_20f"
        freq_sel = freq_CCO164_20f;
        Res_sel = Res_CCO164_20f;
        Vol_sel = Vol_CCO164_20f;
    case "CCO206_0f"
        freq_sel = freq_CCO206_0f;
        Res_sel = Res_CCO206_0f;
        Vol_sel = Vol_CCO206_0f;
    case "CCO206_10f"
        freq_sel = freq_CCO206_10f;
        Res_sel = Res_CCO206_10f;
        Vol_sel = Vol_CCO206_10f;
    case "CCO206_20f"
        freq_sel = freq_CCO206_20f;
        Res_sel = Res_CCO206_20f;
        Vol_sel = Vol_CCO206_20f;
    case "CCO248_0f"
        freq_sel = freq_CCO248_0f;
        Res_sel = Res_CCO248_0f;
        Vol_sel = Vol_CCO248_0f;
    case "CCO248_10f"
        freq_sel = freq_CCO248_10f;
        Res_sel = Res_CCO248_10f;
        Vol_sel = Vol_CCO248_10f;
    case "CCO248_20f"
        freq_sel = freq_CCO248_20f;
        Res_sel = Res_CCO248_20f;
        Vol_sel = Vol_CCO248_20f;
end

freq_sel_N = freq_sel;
freq = spline(x,freq_sel_N,ictrl);
kcco = (spline(x,freq_sel_N,ictrl+delta/2)-spline(x,freq_sel_N,ictrl-delta/2))/delta;
diff_kcco = ((spline(x,freq_sel_N,ictrl+delta/2+gamma/2)-spline(x,freq_sel_N,ictrl-delta/2+gamma/2))/delta-(spline(x,freq_sel_N,ictrl+delta/2-gamma/2)-spline(x,freq_sel_N,ictrl-delta/2-gamma/2))/delta)/gamma;

Res = spline(x,Res_sel,ictrl);
delta = 0.000001;
%Rcco = (f_spline_CCO_vctrl(ictrl+delta/2) - f_spline_CCO_vctrl(ictrl-delta/2))/delta * 1e6;
Vctrl = spline(x, Vol_sel, ictrl);
Rcco = (spline(x, Vol_sel, ictrl+delta/2)-spline(x, Vol_sel, ictrl-delta/2))/delta*1e6;

end

== matlab function CCO_DSM_RDAC_02/MATLAB Function4 ==
  data: ictrl input; freq output; N input; kcco output; CCO_size_num input
%12/07/2021
%0.2uA to 500uA, 15 stages

function [freq, kcco]=f_spline_CCO_all_size_v2(ictrl,N, CCO_size_num)
%%%%%test func
%ictrl = 200;
%N = 31;
%CCO_size = "CCO82_0f";
%%%%%
% CCO_size = ["CCO82_0f","CCO82_10f","CCO82_20f",...
%     "CCO124_0f","CCO124_10f","CCO124_20f",...
%     "CCO164_0f","CCO164_10f","CCO164_20f",...
%     "CCO206_0f","CCO206_10f","CCO206_20f",...
%     "CCO248_0f","CCO248_10f","CCO248_20f"];

delta = 0.0001; % use to calc kvco
gamma = 0.1;

Delay_CCO82 = load('/nethome/kli416/Downloads/VCO/Work/CCO_size_result/Delay_CCO_ring82.txt');
Delay_CCO124 = load('/nethome/kli416/Downloads/VCO/Work/CCO_size_result/Delay_CCO_ring124.txt');
Delay_CCO164 = load('/nethome/kli416/Downloads/VCO/Work/CCO_size_result/Delay_CCO_ring164.txt');
Delay_CCO206 = load('/nethome/kli416/Downloads/VCO/Work/CCO_size_result/Delay_CCO_ring206.txt');
Delay_CCO248 = load('/nethome/kli416/Downloads/VCO/Work/CCO_size_result/Delay_CCO_ring248.txt');
x = [0.2, 0.3, 0.4, 0.5, 0.6, 0.7, 0.8, 0.9, 1.0, 1.1, 1.2, 1.3, 1.4, 1.5, 1.6, 1.7, 1.8, 1.9, 2, 3, 4, 5, 6, 7, 8, 9, 10, 15, 20, 25, 30, 35, 40, 45, 50, 55,  60, 65,  70, 75, 80, 85, 90, 95,  100, 105, 110, 115, 120, 125,  130, 135, 140, 145, 150, 155, 160, 165, 170, 175, 180, 185, 190, 195, 200, 210, 220, 230, 240, 250, 260, 270, 280, 290, 300, 310, 320, 330, 340, 350, 360, 370, 380, 390, 400, 410, 420, 430, 440, 450, 460, 470, 480, 490, 500];
size_x = size(x);
freq_sel = zeros(size_x(2),1);

freq_CCO82_15S_0f = 1./Delay_CCO82(:,1);
freq_CCO82_0f = freq_CCO82_15S_0f*15/N;
freq_CCO82_15S_10f = 1./Delay_CCO82(:,4);
freq_CCO82_10f = freq_CCO82_15S_10f*15/N;
freq_CCO82_15S_20f = 1./Delay_CCO82(:,7);
freq_CCO82_20f = freq_CCO82_15S_20f*15/N;

Res_CCO82_15S_0f = Delay_CCO82(:,3);
Res_CCO82_0f = Res_CCO82_15S_0f;
Res_CCO82_15S_10f = Delay_CCO82(:,6);
Res_CCO82_10f = Res_CCO82_15S_10f;
Res_CCO82_15S_20f = Delay_CCO82(:,9);
Res_CCO82_20f = Res_CCO82_15S_20f;

Vol_CCO82_0f = Delay_CCO82(:,2);
Vol_CCO82_10f = Delay_CCO82(:,5);
Vol_CCO82_20f = Delay_CCO82(:,8);


freq_CCO124_15S_0f = 1./Delay_CCO124(:,1);
freq_CCO124_0f = freq_CCO124_15S_0f*15/N;
freq_CCO124_15S_10f = 1./Delay_CCO124(:,4);
freq_CCO124_10f = freq_CCO124_15S_10f*15/N;
freq_CCO124_15S_20f = 1./Delay_CCO124(:,7);
freq_CCO124_20f = freq_CCO124_15S_20f*15/N;

Res_CCO124_15S_0f = Delay_CCO124(:,3);
Res_CCO124_0f = Res_CCO124_15S_0f;
Res_CCO124_15S_10f = Delay_CCO124(:,6);
Res_CCO124_10f = Res_CCO124_15S_10f;
Res_CCO124_15S_20f = Delay_CCO124(:,9);
Res_CCO124_20f = Res_CCO124_15S_20f;

Vol_CCO124_0f = Delay_CCO124(:,2);
Vol_CCO124_10f = Delay_CCO124(:,5);
Vol_CCO124_20f = Delay_CCO124(:,8);


freq_CCO164_15S_0f = 1./Delay_CCO164(:,1);
freq_CCO164_0f = freq_CCO164_15S_0f*15/N;
freq_CCO164_15S_10f = 1./Delay_CCO164(:,4);
freq_CCO164_10f = freq_CCO164_15S_10f*15/N;
freq_CCO164_15S_20f = 1./Delay_CCO164(:,7);
freq_CCO164_20f = freq_CCO164_15S_20f*15/N;

Res_CCO164_15S_0f = Delay_CCO164(:,3);
Res_CCO164_0f = Res_CCO164_15S_0f;
Res_CCO164_15S_10f = Delay_CCO164(:,6);
Res_CCO164_10f = Res_CCO164_15S_10f;
Res_CCO164_15S_20f = Delay_CCO164(:,9);
Res_CCO164_20f = Res_CCO164_15S_20f;

Vol_CCO164_0f = Delay_CCO164(:,2);
Vol_CCO164_10f = Delay_CCO164(:,5);
Vol_CCO164_20f = Delay_CCO164(:,8);


freq_CCO206_15S_0f = 1./Delay_CCO206(:,1);
freq_CCO206_0f = freq_CCO206_15S_0f*15/N;
freq_CCO206_15S_10f = 1./Delay_CCO206(:,4);
freq_CCO206_10f = freq_CCO206_15S_10f*15/N;
freq_CCO206_15S_20f = 1./Delay_CCO206(:,7);
freq_CCO206_20f = freq_CCO206_15S_20f*15/N;

Res_CCO206_15S_0f = Delay_CCO206(:,3);
Res_CCO206_0f = Res_CCO206_15S_0f;
Res_CCO206_15S_10f = Delay_CCO206(:,6);
Res_CCO206_10f = Res_CCO206_15S_10f;
Res_CCO206_15S_20f = Delay_CCO206(:,9);
Res_CCO206_20f = Res_CCO206_15S_20f;

Vol_CCO206_0f = Delay_CCO206(:,2);
Vol_CCO206_10f = Delay_CCO206(:,5);
Vol_CCO206_20f = Delay_CCO206(:,8);


freq_CCO248_15S_0f = 1./Delay_CCO248(:,1);
freq_CCO248_0f = freq_CCO248_15S_0f*15/N;
freq_CCO248_15S_10f = 1./Delay_CCO248(:,4);
freq_CCO248_10f = freq_CCO248_15S_10f*15/N;
freq_CCO248_15S_20f = 1./Delay_CCO248(:,7);
freq_CCO248_20f = freq_CCO248_15S_20f*15/N;

Res_CCO248_15S_0f = Delay_CCO248(:,3);
Res_CCO248_0f = Res_CCO248_15S_0f;
Res_CCO248_15S_10f = Delay_CCO248(:,6);
Res_CCO248_10f = Res_CCO248_15S_10f;
Res_CCO248_15S_20f = Delay_CCO248(:,9);
Res_CCO248_20f = Res_CCO248_15S_20f;

Vol_CCO248_0f = Delay_CCO248(:,2);
Vol_CCO248_10f = Delay_CCO248(:,5);
Vol_CCO248_20f = Delay_CCO248(:,8);


switch(CCO_size_num)
    case 0%"CCO82_0f"
        freq_sel = freq_CCO82_0f;
        Res_sel = Res_CCO82_0f;
        Vol_sel = Vol_CCO82_0f;
    case 1%"CCO82_10f"
        freq_sel = freq_CCO82_10f;
        Res_sel = Res_CCO82_10f;
        Vol_sel = Vol_CCO82_10f;
    case 2%"CCO82_20f"
        freq_sel = freq_CCO82_20f;
        Res_sel = Res_CCO82_20f;
        Vol_sel = Vol_CCO82_20f;
    case 3%"CCO124_0f"
        freq_sel = freq_CCO124_0f;
        Res_sel = Res_CCO124_0f;
        Vol_sel = Vol_CCO124_0f;
    case 4%"CCO124_10f"
        freq_sel = freq_CCO124_10f;
        Res_sel = Res_CCO124_10f;
        Vol_sel = Vol_CCO124_10f;
    case 5%"CCO124_20f"
        freq_sel = freq_CCO124_20f;
        Res_sel = Res_CCO124_20f;
        Vol_sel = Vol_CCO124_20f;
    case 6%"CCO164_0f"
        freq_sel = freq_CCO164_0f;
        Res_sel = Res_CCO164_0f;
        Vol_sel = Vol_CCO164_0f;
    case 7%"CCO164_10f"
        freq_sel = freq_CCO164_10f;
        Res_sel = Res_CCO164_10f;
        Vol_sel = Vol_CCO164_10f;
    case 8%"CCO164_20f"
        freq_sel = freq_CCO164_20f;
        Res_sel = Res_CCO164_20f;
        Vol_sel = Vol_CCO164_20f;
    case 9%"CCO206_0f"
        freq_sel = freq_CCO206_0f;
        Res_sel = Res_CCO206_0f;
        Vol_sel = Vol_CCO206_0f;
    case 10%"CCO206_10f"
        freq_sel = freq_CCO206_10f;
        Res_sel = Res_CCO206_10f;
        Vol_sel = Vol_CCO206_10f;
    case 11%"CCO206_20f"
        freq_sel = freq_CCO206_20f;
        Res_sel = Res_CCO206_20f;
        Vol_sel = Vol_CCO206_20f;
    case 12%"CCO248_0f"
        freq_sel = freq_CCO248_0f;
        Res_sel = Res_CCO248_0f;
        Vol_sel = Vol_CCO248_0f;
    case 13%"CCO248_10f"
        freq_sel = freq_CCO248_10f;
        Res_sel = Res_CCO248_10f;
        Vol_sel = Vol_CCO248_10f;
    case 14%"CCO248_20f"
        freq_sel = freq_CCO248_20f;
        Res_sel = Res_CCO248_20f;
        Vol_sel = Vol_CCO248_20f;
end

freq_sel_N = freq_sel;
freq = spline(x,freq_sel_N,ictrl);
kcco = (spline(x,freq_sel_N,ictrl+delta/2)-spline(x,freq_sel_N,ictrl-delta/2))/delta;
%diff_kcco = ((spline(x,freq_sel_N,ictrl+delta/2+gamma/2)-spline(x,freq_sel_N,ictrl-delta/2+gamma/2))/delta-(spline(x,freq_sel_N,ictrl+delta/2-gamma/2)-spline(x,freq_sel_N,ictrl-delta/2-gamma/2))/delta)/gamma;

%Res = spline(x,Res_sel,ictrl);
%delta = 0.000001;

%Vctrl = spline(x, Vol_sel, ictrl);
%Rcco = (spline(x, Vol_sel, ictrl+delta/2)-spline(x, Vol_sel, ictrl-delta/2))/delta*1e6;

end

== matlab function CCO_DSM_RDAC_02/Subsystem1/MATLAB Function1 ==
  data: I input; Res output
function Res = Res_CCO(I)
Res = f_spline_CCO_Res_N(I);

end

== matlab function CCO_DSM_RDAC_02/Subsystem1/MATLAB Function2 ==
  data: Res_CCO_fix input; fix_valid input; Res_CCO input; I_out output; R1 input; Ru input; Vin input; count input; DAC_in input; VDD input; Idc input; N input
function I_out = current(Res_CCO_fix, fix_valid, Res_CCO, R1, Ru, Vin, count, DAC_in, VDD, Idc,N)
if (fix_valid == 1)
    %I_out = (Vin-(Idac-compen)*Res*1e-6)/(Res_CCO_fix + Res)*1e6;
    I_out = (Vin/R1*1e6+DAC_in*VDD/Ru*1e6+Idc)/(1+Res_CCO_fix/R1+Res_CCO_fix*N/Ru);
else
    if (count>5)
        I_out = (Vin/R1*1e6+DAC_in*VDD/Ru*1e6+Idc)/(1+Res_CCO/R1+Res_CCO*N/Ru);
    else
        I_out = (Vin/R1*1e6+DAC_in*VDD/Ru*1e6+Idc)/(1+Res_CCO_fix/R1+Res_CCO_fix*N/Ru);
    end
%165e3  47e3  57e3
end
end

== matlab function CCO_DSM_RDAC_02/Subsystem3/MATLAB Function1 ==
  data: I input; Res output
function Res = Res_CCO(I)
Res = f_spline_CCO_Res_N(I);

end
